simulink model "CommSys_300_Bus_Area3"  (Simulink 8.0)
settings: Solver=ode45  StartTime=0.0  StopTime=3800  RelTol=1e-3
libraries: PiccSIM x68
settings Model: Creator=svenda  LastModifiedBy=svenda

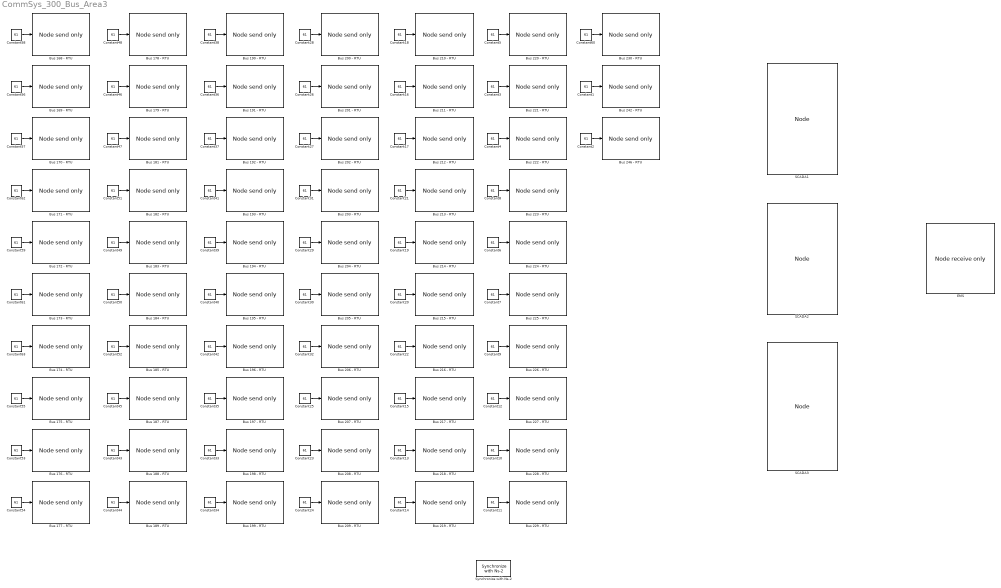
== system CommSys_300_Bus_Area3 ==
  Bus 168 - RTU : PiccSIM/Node send only  ID=0  time_or_seq=Timestamp  sendSchedule=Fixed sampling time  h=2  duty_cycle=1  sendEnable=off  pTypesSend=[10]  sendDataStructure={{'double'}}  externalID=off  sendID={[63]}  coordinates=[0, 0]  IP=NS2_IP
  Bus 169 - RTU : PiccSIM/Node send only  ID=1  time_or_seq=Timestamp  sendSchedule=Fixed sampling time  h=2  duty_cycle=1  sendEnable=off  pTypesSend=[11]  sendDataStructure={{'double'}}  externalID=off  sendID={[63]}  coordinates=[0, 0]  IP=NS2_IP
  Bus 170 - RTU : PiccSIM/Node send only  ID=2  time_or_seq=Timestamp  sendSchedule=Fixed sampling time  h=2  duty_cycle=1  sendEnable=off  pTypesSend=[12]  sendDataStructure={{'double'}}  externalID=off  sendID={[63]}  coordinates=[0, 0]  IP=NS2_IP
  Bus 171 - RTU : PiccSIM/Node send only  ID=3  time_or_seq=Timestamp  sendSchedule=Fixed sampling time  h=2  duty_cycle=1  sendEnable=off  pTypesSend=[13]  sendDataStructure={{'double'}}  externalID=off  sendID={[63]}  coordinates=[0, 0]  IP=NS2_IP
  Bus 172 - RTU : PiccSIM/Node send only  ID=4  time_or_seq=Timestamp  sendSchedule=Fixed sampling time  h=2  duty_cycle=1  sendEnable=off  pTypesSend=[14]  sendDataStructure={{'double'}}  externalID=off  sendID={[63]}  coordinates=[0, 0]  IP=NS2_IP
  Bus 173 - RTU : PiccSIM/Node send only  ID=5  time_or_seq=Timestamp  sendSchedule=Fixed sampling time  h=2  duty_cycle=1  sendEnable=off  pTypesSend=[15]  sendDataStructure={{'double'}}  externalID=off  sendID={[63]}  coordinates=[0, 0]  IP=NS2_IP
  Bus 174 - RTU : PiccSIM/Node send only  ID=6  time_or_seq=Timestamp  sendSchedule=Fixed sampling time  h=2  duty_cycle=1  sendEnable=off  pTypesSend=[16]  sendDataStructure={{'double'}}  externalID=off  sendID={[63]}  coordinates=[0, 0]  IP=NS2_IP
  Bus 175 - RTU : PiccSIM/Node send only  ID=7  time_or_seq=Timestamp  sendSchedule=Fixed sampling time  h=2  duty_cycle=1  sendEnable=off  pTypesSend=[17]  sendDataStructure={{'double'}}  externalID=off  sendID={[63]}  coordinates=[0, 0]  IP=NS2_IP
  Bus 176 - RTU : PiccSIM/Node send only  ID=8  time_or_seq=Timestamp  sendSchedule=Fixed sampling time  h=2  duty_cycle=1  sendEnable=off  pTypesSend=[18]  sendDataStructure={{'double'}}  externalID=off  sendID={[63]}  coordinates=[0, 0]  IP=NS2_IP
  Bus 177 - RTU : PiccSIM/Node send only  ID=9  time_or_seq=Timestamp  sendSchedule=Fixed sampling time  h=2  duty_cycle=1  sendEnable=off  pTypesSend=[19]  sendDataStructure={{'double'}}  externalID=off  sendID={[63]}  coordinates=[0, 0]  IP=NS2_IP
  Bus 178 - RTU : PiccSIM/Node send only  ID=10  time_or_seq=Timestamp  sendSchedule=Fixed sampling time  h=2  duty_cycle=1  sendEnable=off  pTypesSend=[110]  sendDataStructure={{'double'}}  externalID=off  sendID={[63]}  coordinates=[0, 0]  IP=NS2_IP
  Bus 179 - RTU : PiccSIM/Node send only  ID=11  time_or_seq=Timestamp  sendSchedule=Fixed sampling time  h=2  duty_cycle=1  sendEnable=off  pTypesSend=[111]  sendDataStructure={{'double'}}  externalID=off  sendID={[63]}  coordinates=[0, 0]  IP=NS2_IP
  Bus 181 - RTU : PiccSIM/Node send only  ID=12  time_or_seq=Timestamp  sendSchedule=Fixed sampling time  h=2  duty_cycle=1  sendEnable=off  pTypesSend=[112]  sendDataStructure={{'double'}}  externalID=off  sendID={[63]}  coordinates=[0, 0]  IP=NS2_IP
  Bus 182 - RTU : PiccSIM/Node send only  ID=13  time_or_seq=Timestamp  sendSchedule=Fixed sampling time  h=2  duty_cycle=1  sendEnable=off  pTypesSend=[113]  sendDataStructure={{'double'}}  externalID=off  sendID={[63]}  coordinates=[0, 0]  IP=NS2_IP
  Bus 183 - RTU : PiccSIM/Node send only  ID=14  time_or_seq=Timestamp  sendSchedule=Fixed sampling time  h=2  duty_cycle=1  sendEnable=off  pTypesSend=[114]  sendDataStructure={{'double'}}  externalID=off  sendID={[63]}  coordinates=[0, 0]  IP=NS2_IP
  Bus 184 - RTU : PiccSIM/Node send only  ID=15  time_or_seq=Timestamp  sendSchedule=Fixed sampling time  h=2  duty_cycle=1  sendEnable=off  pTypesSend=[115]  sendDataStructure={{'double'}}  externalID=off  sendID={[63]}  coordinates=[0, 0]  IP=NS2_IP
  Bus 185 - RTU : PiccSIM/Node send only  ID=16  time_or_seq=Timestamp  sendSchedule=Fixed sampling time  h=2  duty_cycle=1  sendEnable=off  pTypesSend=[116]  sendDataStructure={{'double'}}  externalID=off  sendID={[63]}  coordinates=[0, 0]  IP=NS2_IP
  Bus 187 - RTU : PiccSIM/Node send only  ID=17  time_or_seq=Timestamp  sendSchedule=Fixed sampling time  h=2  duty_cycle=1  sendEnable=off  pTypesSend=[117]  sendDataStructure={{'double'}}  externalID=off  sendID={[63]}  coordinates=[0, 0]  IP=NS2_IP
  Bus 188 - RTU : PiccSIM/Node send only  ID=18  time_or_seq=Timestamp  sendSchedule=Fixed sampling time  h=2  duty_cycle=1  sendEnable=off  pTypesSend=[118]  sendDataStructure={{'double'}}  externalID=off  sendID={[63]}  coordinates=[0, 0]  IP=NS2_IP
  Bus 189 - RTU : PiccSIM/Node send only  ID=19  time_or_seq=Timestamp  sendSchedule=Fixed sampling time  h=2  duty_cycle=1  sendEnable=off  pTypesSend=[119]  sendDataStructure={{'double'}}  externalID=off  sendID={[63]}  coordinates=[0, 0]  IP=NS2_IP
  Bus 190 - RTU : PiccSIM/Node send only  ID=20  time_or_seq=Timestamp  sendSchedule=Fixed sampling time  h=2  duty_cycle=1  sendEnable=off  pTypesSend=[120]  sendDataStructure={{'double'}}  externalID=off  sendID={[64]}  coordinates=[0, 0]  IP=NS2_IP
  Bus 191 - RTU : PiccSIM/Node send only  ID=21  time_or_seq=Timestamp  sendSchedule=Fixed sampling time  h=2  duty_cycle=1  sendEnable=off  pTypesSend=[121]  sendDataStructure={{'double'}}  externalID=off  sendID={[64]}  coordinates=[0, 0]  IP=NS2_IP
  Bus 192 - RTU : PiccSIM/Node send only  ID=22  time_or_seq=Timestamp  sendSchedule=Fixed sampling time  h=2  duty_cycle=1  sendEnable=off  pTypesSend=[122]  sendDataStructure={{'double'}}  externalID=off  sendID={[64]}  coordinates=[0, 0]  IP=NS2_IP
  Bus 193 - RTU : PiccSIM/Node send only  ID=23  time_or_seq=Timestamp  sendSchedule=Fixed sampling time  h=2  duty_cycle=1  sendEnable=off  pTypesSend=[123]  sendDataStructure={{'double'}}  externalID=off  sendID={[64]}  coordinates=[0, 0]  IP=NS2_IP
  Bus 194 - RTU : PiccSIM/Node send only  ID=24  time_or_seq=Timestamp  sendSchedule=Fixed sampling time  h=2  duty_cycle=1  sendEnable=off  pTypesSend=[124]  sendDataStructure={{'double'}}  externalID=off  sendID={[64]}  coordinates=[0, 0]  IP=NS2_IP
  Bus 195 - RTU : PiccSIM/Node send only  ID=25  time_or_seq=Timestamp  sendSchedule=Fixed sampling time  h=2  duty_cycle=1  sendEnable=off  pTypesSend=[125]  sendDataStructure={{'double'}}  externalID=off  sendID={[64]}  coordinates=[0, 0]  IP=NS2_IP
  Bus 196 - RTU : PiccSIM/Node send only  ID=26  time_or_seq=Timestamp  sendSchedule=Fixed sampling time  h=2  duty_cycle=1  sendEnable=off  pTypesSend=[126]  sendDataStructure={{'double'}}  externalID=off  sendID={[64]}  coordinates=[0, 0]  IP=NS2_IP
  Bus 197 - RTU : PiccSIM/Node send only  ID=27  time_or_seq=Timestamp  sendSchedule=Fixed sampling time  h=2  duty_cycle=1  sendEnable=off  pTypesSend=[127]  sendDataStructure={{'double'}}  externalID=off  sendID={[64]}  coordinates=[0, 0]  IP=NS2_IP
  Bus 198 - RTU : PiccSIM/Node send only  ID=28  time_or_seq=Timestamp  sendSchedule=Fixed sampling time  h=2  duty_cycle=1  sendEnable=off  pTypesSend=[128]  sendDataStructure={{'double'}}  externalID=off  sendID={[64]}  coordinates=[0, 0]  IP=NS2_IP
  Bus 199 - RTU : PiccSIM/Node send only  ID=29  time_or_seq=Timestamp  sendSchedule=Fixed sampling time  h=2  duty_cycle=1  sendEnable=off  pTypesSend=[129]  sendDataStructure={{'double'}}  externalID=off  sendID={[64]}  coordinates=[0, 0]  IP=NS2_IP
  Bus 200 - RTU : PiccSIM/Node send only  ID=30  time_or_seq=Timestamp  sendSchedule=Fixed sampling time  h=2  duty_cycle=1  sendEnable=off  pTypesSend=[130]  sendDataStructure={{'double'}}  externalID=off  sendID={[64]}  coordinates=[0, 0]  IP=NS2_IP
  Bus 201 - RTU : PiccSIM/Node send only  ID=31  time_or_seq=Timestamp  sendSchedule=Fixed sampling time  h=2  duty_cycle=1  sendEnable=off  pTypesSend=[131]  sendDataStructure={{'double'}}  externalID=off  sendID={[64]}  coordinates=[0, 0]  IP=NS2_IP
  Bus 202 - RTU : PiccSIM/Node send only  ID=32  time_or_seq=Timestamp  sendSchedule=Fixed sampling time  h=2  duty_cycle=1  sendEnable=off  pTypesSend=[132]  sendDataStructure={{'double'}}  externalID=off  sendID={[64]}  coordinates=[0, 0]  IP=NS2_IP
  Bus 203 - RTU : PiccSIM/Node send only  ID=33  time_or_seq=Timestamp  sendSchedule=Fixed sampling time  h=2  duty_cycle=1  sendEnable=off  pTypesSend=[133]  sendDataStructure={{'double'}}  externalID=off  sendID={[64]}  coordinates=[0, 0]  IP=NS2_IP
  Bus 204 - RTU : PiccSIM/Node send only  ID=34  time_or_seq=Timestamp  sendSchedule=Fixed sampling time  h=2  duty_cycle=1  sendEnable=off  pTypesSend=[134]  sendDataStructure={{'double'}}  externalID=off  sendID={[64]}  coordinates=[0, 0]  IP=NS2_IP
  Bus 205 - RTU : PiccSIM/Node send only  ID=35  time_or_seq=Timestamp  sendSchedule=Fixed sampling time  h=2  duty_cycle=1  sendEnable=off  pTypesSend=[135]  sendDataStructure={{'double'}}  externalID=off  sendID={[64]}  coordinates=[0, 0]  IP=NS2_IP
  Bus 206 - RTU : PiccSIM/Node send only  ID=36  time_or_seq=Timestamp  sendSchedule=Fixed sampling time  h=2  duty_cycle=1  sendEnable=off  pTypesSend=[136]  sendDataStructure={{'double'}}  externalID=off  sendID={[64]}  coordinates=[0, 0]  IP=NS2_IP
  Bus 207 - RTU : PiccSIM/Node send only  ID=37  time_or_seq=Timestamp  sendSchedule=Fixed sampling time  h=2  duty_cycle=1  sendEnable=off  pTypesSend=[137]  sendDataStructure={{'double'}}  externalID=off  sendID={[64]}  coordinates=[0, 0]  IP=NS2_IP
  Bus 208 - RTU : PiccSIM/Node send only  ID=38  time_or_seq=Timestamp  sendSchedule=Fixed sampling time  h=2  duty_cycle=1  sendEnable=off  pTypesSend=[138]  sendDataStructure={{'double'}}  externalID=off  sendID={[64]}  coordinates=[0, 0]  IP=NS2_IP
  Bus 209 - RTU : PiccSIM/Node send only  ID=39  time_or_seq=Timestamp  sendSchedule=Fixed sampling time  h=2  duty_cycle=1  sendEnable=off  pTypesSend=[139]  sendDataStructure={{'double'}}  externalID=off  sendID={[64]}  coordinates=[0, 0]  IP=NS2_IP
  Bus 210 - RTU : PiccSIM/Node send only  ID=40  time_or_seq=Timestamp  sendSchedule=Fixed sampling time  h=2  duty_cycle=1  sendEnable=off  pTypesSend=[140]  sendDataStructure={{'double'}}  externalID=off  sendID={[65]}  coordinates=[0, 0]  IP=NS2_IP
  Bus 211 - RTU : PiccSIM/Node send only  ID=41  time_or_seq=Timestamp  sendSchedule=Fixed sampling time  h=2  duty_cycle=1  sendEnable=off  pTypesSend=[141]  sendDataStructure={{'double'}}  externalID=off  sendID={[65]}  coordinates=[0, 0]  IP=NS2_IP
  Bus 212 - RTU : PiccSIM/Node send only  ID=42  time_or_seq=Timestamp  sendSchedule=Fixed sampling time  h=2  duty_cycle=1  sendEnable=off  pTypesSend=[142]  sendDataStructure={{'double'}}  externalID=off  sendID={[65]}  coordinates=[0, 0]  IP=NS2_IP
  Bus 213 - RTU : PiccSIM/Node send only  ID=43  time_or_seq=Timestamp  sendSchedule=Fixed sampling time  h=2  duty_cycle=1  sendEnable=off  pTypesSend=[143]  sendDataStructure={{'double'}}  externalID=off  sendID={[65]}  coordinates=[0, 0]  IP=NS2_IP
  Bus 214 - RTU : PiccSIM/Node send only  ID=44  time_or_seq=Timestamp  sendSchedule=Fixed sampling time  h=2  duty_cycle=1  sendEnable=off  pTypesSend=[144]  sendDataStructure={{'double'}}  externalID=off  sendID={[65]}  coordinates=[0, 0]  IP=NS2_IP
  Bus 215 - RTU : PiccSIM/Node send only  ID=45  time_or_seq=Timestamp  sendSchedule=Fixed sampling time  h=2  duty_cycle=1  sendEnable=off  pTypesSend=[145]  sendDataStructure={{'double'}}  externalID=off  sendID={[65]}  coordinates=[0, 0]  IP=NS2_IP
  Bus 216 - RTU : PiccSIM/Node send only  ID=46  time_or_seq=Timestamp  sendSchedule=Fixed sampling time  h=2  duty_cycle=1  sendEnable=off  pTypesSend=[146]  sendDataStructure={{'double'}}  externalID=off  sendID={[65]}  coordinates=[0, 0]  IP=NS2_IP
  Bus 217 - RTU : PiccSIM/Node send only  ID=47  time_or_seq=Timestamp  sendSchedule=Fixed sampling time  h=2  duty_cycle=1  sendEnable=off  pTypesSend=[147]  sendDataStructure={{'double'}}  externalID=off  sendID={[65]}  coordinates=[0, 0]  IP=NS2_IP
  Bus 218 - RTU : PiccSIM/Node send only  ID=48  time_or_seq=Timestamp  sendSchedule=Fixed sampling time  h=2  duty_cycle=1  sendEnable=off  pTypesSend=[148]  sendDataStructure={{'double'}}  externalID=off  sendID={[65]}  coordinates=[0, 0]  IP=NS2_IP
  Bus 219 - RTU : PiccSIM/Node send only  ID=49  time_or_seq=Timestamp  sendSchedule=Fixed sampling time  h=2  duty_cycle=1  sendEnable=off  pTypesSend=[149]  sendDataStructure={{'double'}}  externalID=off  sendID={[65]}  coordinates=[0, 0]  IP=NS2_IP
  Bus 220 - RTU : PiccSIM/Node send only  ID=50  time_or_seq=Timestamp  sendSchedule=Fixed sampling time  h=2  duty_cycle=1  sendEnable=off  pTypesSend=[150]  sendDataStructure={{'double'}}  externalID=off  sendID={[65]}  coordinates=[0, 0]  IP=NS2_IP
  Bus 221 - RTU : PiccSIM/Node send only  ID=51  time_or_seq=Timestamp  sendSchedule=Fixed sampling time  h=2  duty_cycle=1  sendEnable=off  pTypesSend=[151]  sendDataStructure={{'double'}}  externalID=off  sendID={[65]}  coordinates=[0, 0]  IP=NS2_IP
  Bus 222 - RTU : PiccSIM/Node send only  ID=52  time_or_seq=Timestamp  sendSchedule=Fixed sampling time  h=2  duty_cycle=1  sendEnable=off  pTypesSend=[152]  sendDataStructure={{'double'}}  externalID=off  sendID={[65]}  coordinates=[0, 0]  IP=NS2_IP
  Bus 223 - RTU : PiccSIM/Node send only  ID=53  time_or_seq=Timestamp  sendSchedule=Fixed sampling time  h=2  duty_cycle=1  sendEnable=off  pTypesSend=[153]  sendDataStructure={{'double'}}  externalID=off  sendID={[65]}  coordinates=[0, 0]  IP=NS2_IP
  Bus 224 - RTU : PiccSIM/Node send only  ID=54  time_or_seq=Timestamp  sendSchedule=Fixed sampling time  h=2  duty_cycle=1  sendEnable=off  pTypesSend=[154]  sendDataStructure={{'double'}}  externalID=off  sendID={[65]}  coordinates=[0, 0]  IP=NS2_IP
  Bus 225 - RTU : PiccSIM/Node send only  ID=55  time_or_seq=Timestamp  sendSchedule=Fixed sampling time  h=2  duty_cycle=1  sendEnable=off  pTypesSend=[155]  sendDataStructure={{'double'}}  externalID=off  sendID={[65]}  coordinates=[0, 0]  IP=NS2_IP
  Bus 226 - RTU : PiccSIM/Node send only  ID=56  time_or_seq=Timestamp  sendSchedule=Fixed sampling time  h=2  duty_cycle=1  sendEnable=off  pTypesSend=[156]  sendDataStructure={{'double'}}  externalID=off  sendID={[65]}  coordinates=[0, 0]  IP=NS2_IP
  Bus 227 - RTU : PiccSIM/Node send only  ID=57  time_or_seq=Timestamp  sendSchedule=Fixed sampling time  h=2  duty_cycle=1  sendEnable=off  pTypesSend=[157]  sendDataStructure={{'double'}}  externalID=off  sendID={[65]}  coordinates=[0, 0]  IP=NS2_IP
  Bus 228 - RTU : PiccSIM/Node send only  ID=58  time_or_seq=Timestamp  sendSchedule=Fixed sampling time  h=2  duty_cycle=1  sendEnable=off  pTypesSend=[158]  sendDataStructure={{'double'}}  externalID=off  sendID={[65]}  coordinates=[0, 0]  IP=NS2_IP
  Bus 229 - RTU : PiccSIM/Node send only  ID=59  time_or_seq=Timestamp  sendSchedule=Fixed sampling time  h=2  duty_cycle=1  sendEnable=off  pTypesSend=[159]  sendDataStructure={{'double'}}  externalID=off  sendID={[65]}  coordinates=[0, 0]  IP=NS2_IP
  Bus 230 - RTU : PiccSIM/Node send only  ID=60  time_or_seq=Timestamp  sendSchedule=Fixed sampling time  h=2  duty_cycle=1  sendEnable=off  pTypesSend=[160]  sendDataStructure={{'double'}}  externalID=off  sendID={[65]}  coordinates=[0, 0]  IP=NS2_IP
  Bus 242 - RTU : PiccSIM/Node send only  ID=61  time_or_seq=Timestamp  sendSchedule=Fixed sampling time  h=2  duty_cycle=1  sendEnable=off  pTypesSend=[161]  sendDataStructure={{'double'}}  externalID=off  sendID={[65]}  coordinates=[0, 0]  IP=NS2_IP
  Bus 246 - RTU : PiccSIM/Node send only  ID=62  time_or_seq=Timestamp  sendSchedule=Fixed sampling time  h=2  duty_cycle=1  sendEnable=off  pTypesSend=[162]  sendDataStructure={{'double'}}  externalID=off  sendID={[65]}  coordinates=[0, 0]  IP=NS2_IP
  Constant{1..63} (63 alike) : Constant  Value=61
  EMS : PiccSIM/Node receive only  ID=66  pTypes=[163, 164, 165]  receiveDataLengths={{[1]}, {[1]}, {[1]}}  receiveDataStructure={{'double'}, {'double'}, {'double'}}  recFrom={[63], [64], [65]}  coordinates=[0, 0]  IP=NS2_IP
  SCADA1 : PiccSIM/Node  ID=63  time_or_seq=Timestamp  sendSchedule=Fixed sampling time  h=2  duty_cycle=1  sendEnable=off  pTypesSend=[163]  sendDataStructure={{'double'}}  externalID=off  sendID={[66]}  pTypes=[10, 11, 12, 13, 14, 15, 16, 17, 18, 19, 110, 111, 112, 113, 114, 115, 116, 117, 118, 119]  receiveDataLengths={{[1]}, {[1]}, {[1]}, {[1]}, {[1]}, {[1]}, {[1]}, {[1]}, {[1]}, {[1]}, {[1]}, {[1]}, {[1]}, {[1]}, {[1]}, {[1]}, {[1]}, {[1]}, {[1]}, {[1]}}  receiveDataStructure={{'double'}, {'double'}, {'double'}, {'double'}, {'double'}, {'double'}, {'double'}, {'double'}, {'double'}, {'double'}, {'double'}, {'double'}, {'double'}, {'double'}, {'double'}, {'double'}, {'double'}, {'double'}, {'double'}, {'double'}}  recFrom={[0], [1], [2], [3], [4], [5], [6], [7], [8], [9], [10], [11], [12], [13], [14], [15], [16], [17], [18], [19]}  coordinates=[0, 0]  IP=NS2_IP
  SCADA2 : PiccSIM/Node  ID=64  time_or_seq=Timestamp  sendSchedule=Fixed sampling time  h=2  duty_cycle=1  sendEnable=off  pTypesSend=[164]  sendDataStructure={{'double'}}  externalID=off  sendID={[66]}  pTypes=[120, 121, 122, 123, 124, 125, 126, 127, 128, 129, 130, 131, 132, 133, 134, 135, 136, 137, 138, 139]  receiveDataLengths={{[1]}, {[1]}, {[1]}, {[1]}, {[1]}, {[1]}, {[1]}, {[1]}, {[1]}, {[1]}, {[1]}, {[1]}, {[1]}, {[1]}, {[1]}, {[1]}, {[1]}, {[1]}, {[1]}, {[1]}}  receiveDataStructure={{'double'}, {'double'}, {'double'}, {'double'}, {'double'}, {'double'}, {'double'}, {'double'}, {'double'}, {'double'}, {'double'}, {'double'}, {'double'}, {'double'}, {'double'}, {'double'}, {'double'}, {'double'}, {'double'}, {'double'}}  recFrom={[20], [21], [22], [23], [24], [25], [26], [27], [28], [29], [30], [31], [32], [33], [34], [35], [36], [37], [38], [39]}  coordinates=[0, 0]  IP=NS2_IP
  SCADA3 : PiccSIM/Node  ID=65  time_or_seq=Timestamp  sendSchedule=Fixed sampling time  h=2  duty_cycle=1  sendEnable=off  pTypesSend=[165]  sendDataStructure={{'double'}}  externalID=off  sendID={[66]}  pTypes=[140, 141, 142, 143, 144, 145, 146, 147, 148, 149, 150, 151, 152, 153, 154, 155, 156, 157, 158, 159, 160, 161, 162]  receiveDataLengths={{[1]}, {[1]}, {[1]}, {[1]}, {[1]}, {[1]}, {[1]}, {[1]}, {[1]}, {[1]}, {[1]}, {[1]}, {[1]}, {[1]}, {[1]}, {[1]}, {[1]}, {[1]}, {[1]}, {[1]}, {[1]}, {[1]}, {[1]}}  receiveDataStructure={{'double'}, {'double'}, {'double'}, {'double'}, {'double'}, {'double'}, {'double'}, {'double'}, {'double'}, {'double'}, {'double'}, {'double'}, {'double'}, {'double'}, {'double'}, {'double'}, {'double'}, {'double'}, {'double'}, {'double'}, {'double'}, {'double'}, {'double'}}  recFrom={[40], [41], [42], [43], [44], [45], [46], [47], [48], [49], [50], [51], [52], [53], [54], [55], [56], [57], [58], [59], [60], [61], [62]}  coordinates=[0, 0]  IP=NS2_IP
  Synchronize with Ns-2 : PiccSIM/Synchronize with Ns-2  Priority=100000  c=1  port=23201  IP=NS2_IP
  wires:
  Constant60/1 -> Bus 230 - RTU/1
  Constant1/1 -> Bus 242 - RTU/1
  Constant2/1 -> Bus 246 - RTU/1
  Constant5/1 -> Bus 220 - RTU/1
  Constant3/1 -> Bus 221 - RTU/1
  Constant4/1 -> Bus 222 - RTU/1
  Constant8/1 -> Bus 223 - RTU/1
  Constant6/1 -> Bus 224 - RTU/1
  Constant7/1 -> Bus 225 - RTU/1
  Constant9/1 -> Bus 226 - RTU/1
  Constant12/1 -> Bus 227 - RTU/1
  Constant10/1 -> Bus 228 - RTU/1
  Constant11/1 -> Bus 229 - RTU/1
  Constant18/1 -> Bus 210 - RTU/1
  Constant16/1 -> Bus 211 - RTU/1
  Constant17/1 -> Bus 212 - RTU/1
  Constant21/1 -> Bus 213 - RTU/1
  Constant19/1 -> Bus 214 - RTU/1
  Constant20/1 -> Bus 215 - RTU/1
  Constant22/1 -> Bus 216 - RTU/1
  Constant15/1 -> Bus 217 - RTU/1
  Constant13/1 -> Bus 218 - RTU/1
  Constant14/1 -> Bus 219 - RTU/1
  Constant28/1 -> Bus 200 - RTU/1
  Constant26/1 -> Bus 201 - RTU/1
  Constant27/1 -> Bus 202 - RTU/1
  Constant31/1 -> Bus 203 - RTU/1
  Constant29/1 -> Bus 204 - RTU/1
  Constant30/1 -> Bus 205 - RTU/1
  Constant32/1 -> Bus 206 - RTU/1
  Constant25/1 -> Bus 207 - RTU/1
  Constant23/1 -> Bus 208 - RTU/1
  Constant24/1 -> Bus 209 - RTU/1
  Constant38/1 -> Bus 190 - RTU/1
  Constant36/1 -> Bus 191 - RTU/1
  Constant37/1 -> Bus 192 - RTU/1
  Constant41/1 -> Bus 193 - RTU/1
  Constant39/1 -> Bus 194 - RTU/1
  Constant40/1 -> Bus 195 - RTU/1
  Constant42/1 -> Bus 196 - RTU/1
  Constant35/1 -> Bus 197 - RTU/1
  Constant33/1 -> Bus 198 - RTU/1
  Constant34/1 -> Bus 199 - RTU/1
  Constant48/1 -> Bus 178 - RTU/1
  Constant46/1 -> Bus 179 - RTU/1
  Constant47/1 -> Bus 181 - RTU/1
  Constant51/1 -> Bus 182 - RTU/1
  Constant49/1 -> Bus 183 - RTU/1
  Constant50/1 -> Bus 184 - RTU/1
  Constant52/1 -> Bus 185 - RTU/1
  Constant45/1 -> Bus 187 - RTU/1
  Constant43/1 -> Bus 188 - RTU/1
  Constant44/1 -> Bus 189 - RTU/1
  Constant58/1 -> Bus 168 - RTU/1
  Constant56/1 -> Bus 169 - RTU/1
  Constant57/1 -> Bus 170 - RTU/1
  Constant62/1 -> Bus 171 - RTU/1
  Constant59/1 -> Bus 172 - RTU/1
  Constant61/1 -> Bus 173 - RTU/1
  Constant63/1 -> Bus 174 - RTU/1
  Constant55/1 -> Bus 175 - RTU/1
  Constant53/1 -> Bus 176 - RTU/1
  Constant54/1 -> Bus 177 - RTU/1
